simulink model "lookupTableDynamic_TestGen2"  (R2017b)
settings: Solver=FixedStepDiscrete  StartTime=0.0  StopTime=10.0  RelTol=1e-3
libraries: simulink x1
settings Model: Creator=ktrinh  LastModifiedBy=ktrinh
settings DebuggingCC: ParameterOverflowMsg=none

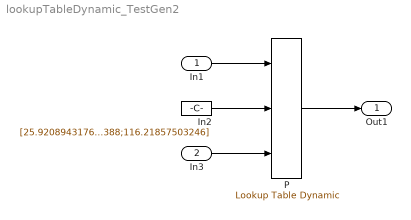
== system lookupTableDynamic_TestGen2 ==
  In1 : Inport  OutMin=23.9209  OutMax=118.2186  OutDataTypeStr=single  PortDimensions=3
  In3 : Inport  Port=2  PortDimensions=5
  In2 : Constant  Value=[25.9208943176654;43.490025525633;72.9782375689138;85.3979753212388;116.21857503246]  OutDataTypeStr=single
  P : simulink/Lookup Tables/Lookup Table Dynamic  LookUpMeth=Interpolation-Extrapolation  OutDataType=fixdt('single')  OutScaling=[]  OutputDataTypeScalingMode=Specify via dialog  OutDataTypeStr=single  DoSatur=off
      settings: SourceProductName=Simulink
  Out1 : Outport
  wires:
  In1/1 -> P/1
  In2/1 -> P/2
  In3/1 -> P/3
  P/1 -> Out1/1
